simulink model "Power_Model_Official_Pars"  (R2023a)
settings: Solver=ode23t  StartTime=0.0  StopTime=1000  FixedStep=0.01  MaxStep=0.01  RelTol=1e-3  AbsTol=1e-3
values from neighbouring files (symbols this model uses):
  anode_tube_D = 0.01    [fuel_cell_battery_par.mat]
  cathode_tube_D = 0.05    [fuel_cell_battery_par.mat]
  comp_rpm_TLU = [0 1800 3600]    [fuel_cell_battery_par.mat]
  coolant_num_layers = 20    [fuel_cell_battery_par.mat]
  coolant_num_passes = 12    [fuel_cell_battery_par.mat]
  coolant_tube_D = 0.05    [fuel_cell_battery_par.mat]
  coolant_w_channels = 1    [fuel_cell_battery_par.mat]
  env_p = 0.101325    [fuel_cell_battery_par.mat]
  env_T = 20    [fuel_cell_battery_par.mat]
  env_yH20 = 0.0115436377169    [fuel_cell_battery_par.mat]
  env_yO2 = 0.21    [fuel_cell_battery_par.mat]
  radiator_air_area_fins = 11.5625    [fuel_cell_battery_par.mat]
  radiator_air_area_primary = 1.223125    [fuel_cell_battery_par.mat]
  radiator_eta_fin = 0.7    [fuel_cell_battery_par.mat]
  radiator_N_tubes = 25    [fuel_cell_battery_par.mat]
  radiator_rho = 2700    [fuel_cell_battery_par.mat]
  radiator_t_wall = 0.0001    [fuel_cell_battery_par.mat]
  radiator_tube_H = 0.0015    [fuel_cell_battery_par.mat]
  radiator_W = 0.025    [fuel_cell_battery_par.mat]
  stack_area = 280    [fuel_cell_battery_par.mat]
  stack_iL = 1.4    [fuel_cell_battery_par.mat]
  stack_mea_rho = 1800    [fuel_cell_battery_par.mat]
  stack_num_cells = 400    [fuel_cell_battery_par.mat]
  stack_num_channels = 8    [fuel_cell_battery_par.mat]
  stack_t_gdl = 250    [fuel_cell_battery_par.mat]
  stack_t_membrane = 125    [fuel_cell_battery_par.mat]
  stack_w_channels = 1    [fuel_cell_battery_par.mat]
undefined symbols (not defined in the file or in its folder): Bat, f_fc_auxpower, f_fc_currcmd_bpt, f_fc_h2flow, f_fc_heatflow, f_fc_tmpcmd_bpt, f_fc_voltage, Mot, N2_T
libraries: fl_lib x170, nesl_utility x78, FuelCell_lib x32, simulink x5, slpidlib x4, ee_lib x3, autolibshared x1, batteryecm_lib x1, simulink_extras x1
(part 4 of 9)

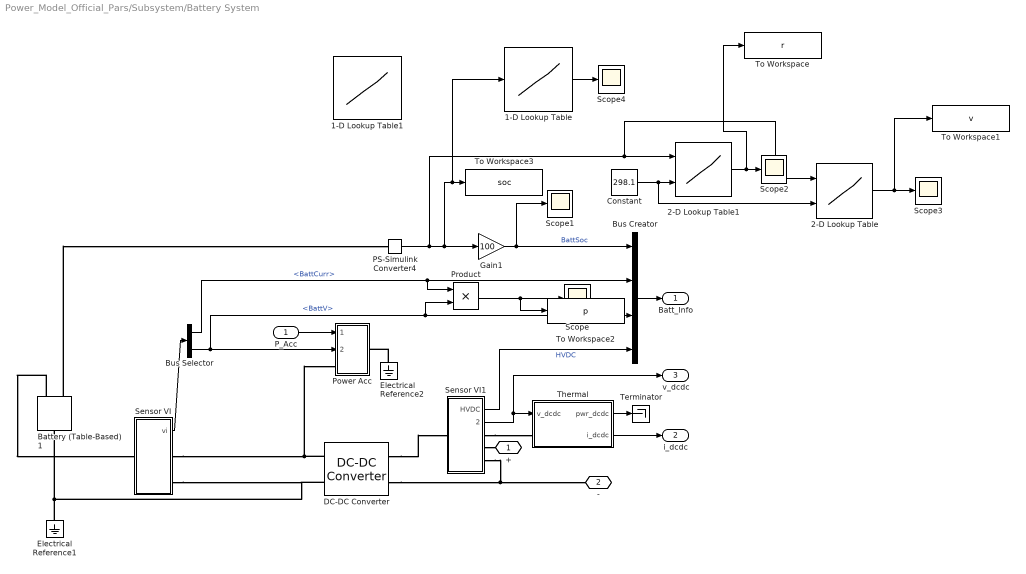
== system Power_Model_Official_Pars/Subsystem/Battery System ==
  P_Acc : Inport
  1-D Lookup Table : Lookup_n-D  NumberOfTableDimensions=1  BreakpointsForDimension1=|  IndexSearchMethod=Linear search  Table=|  ExtrapMethod=Clip  UseLastTableValue=on  InternalRulePriority=Speed  RndMeth=Simplest
      BreakpointsForDimension1=|
      | [0.200266196912653
      | 0.208703993443662
      | 0.217082158618762
      | 0.225401147932810
      | 0.233661407473458
      | 0.241863374201597
      | 0.250007476220565
      | 0.258094133034692
      | 0.266123755797699
      | 0.274096747551458
      | 0.282013503455571
      | 0.289874411008216
      | 0.297679850258674
      | 0.305430194011883
      | 0.313125808025436
      | 0.320767051200107
      | 0.328354275760887
      | 0.335887827433726
      | 0.343368045619003
      | 0.350795263562739
      | 0.358169809006629
      | 0.365492002225901
      | 0.372762157540920
      | 0.379980604257750
      | 0.387147663219995
      | 0.394263583481661
      | 0.401328845877270
      | 0.408344807259339
      | 0.415312528633151
      | 0.422232177852414
      | 0.429103921869992
      | 0.435927926732909
      | 0.442704357577685
      | 0.449433378625998
      | 0.456115153180668
      | 0.462749843621933
      | 0.469337611404045
      | 0.475878617052130
      | 0.482373020159354
      | 0.488820979384337
      | 0.495222652448848
      | 0.501578196135747
      | 0.507887766287174
      | 0.514151517802985
      | 0.520369604639409
      | 0.526542179807939
      | 0.532669395374436
      | 0.538751402458431
      | 0.544788351232696
      | 0.550780390922972
      | 0.556727669807170
      | 0.562630335217596
      | 0.568488533530473
      | 0.574302410199744
      | 0.580072109717100
      | 0.585797772346718
      | 0.591479540262522
      | 0.597117565243885
      | 0.602710710150421
      | 0.608256553325338
      | 0.613754051013394
      | 0.619203525910865
      | 0.624605294684209
      | 0.629959668123070
      | 0.635266951288040
      | 0.640527443653388
      | 0.645741439244992
      | 0.650909226773650
      | 0.656031089763978
      | 0.661107306679072
      | 0.666138151041100
      | 0.671123891547999
      | 0.676064792186425
      | 0.680961112341104
      | 0.685813106900738
      | 0.690621026360585
      | 0.695385116921850
      | 0.700105620588011
      | 0.704782775258189
      | 0.709416814817689
      | 0.714007969225799
      | 0.718556464600965
      | 0.723062523303430
      | 0.727526364015437
      | 0.731948201819075
      | 0.736328248271866
      | 0.740666711480160
      | 0.744963796170435
      | 0.749219703758548
      | 0.753434632417049
      | 0.757608777140570
      | 0.761742329809332
      | 0.765835479251445
      | 0.769888411303126
      | 0.773901308859363
      | 0.777874351956835
      | 0.781807718120983
      | 0.785701580794767
      | 0.789556112063642
      | 0.793371492233416
      | 0.797147876670597
      | 0.800885457679393
      | 0.804584556002125
      | 0.808245419955624
      | 0.811868165288415
      | 0.815452907369891
      | 0.818999761410582
      | 0.822508841965610
      | 0.825980262919708
      | 0.829414137942514
      | 0.832810580234303
      | 0.836169702509582
      | 0.839491616981221
      | 0.842776435345101
      | 0.846024268765268
      | 0.849235227859599
      | 0.852409422685936
      | 0.855546962728712
      | 0.858647956886038
      | 0.861712513457244
      | 0.864740740130864
      | 0.867732743973058
      | 0.870688631416451
      | 0.873608508249394
      | 0.876492479605619
      | 0.879340649954288
      | 0.882153123090427
      | 0.884930002125727
      | 0.887671389479714
      | 0.890377386871260
      | 0.893048095310450
      | 0.895683615090770
      | 0.898284045781626
      | 0.900849486221171
      | 0.903380034509446
      | 0.905875788001805
      | 0.908336843302639
      | 0.910763296259371
      | 0.913155241956721
      | 0.915512774711237
      | 0.917835988066077
      | 0.920124974786031
      | 0.922379826852788
      | 0.924600635460429
      | 0.926787491011139
      | 0.928940483111134
      | 0.931059700566797
      | 0.933145231381011
      | 0.935197162749684
      | 0.937215581058461
      | 0.939200571879608
      | 0.941152219969077
      | 0.943070609263730
      | 0.944955822878720
      | 0.946807943105026
      | 0.948627051407141
      | 0.950413228420884
      | 0.952166553951363
      | 0.953887106971052
      | 0.955574965618005
      | 0.957230207194170
      | 0.958852908163831
      | 0.960443144152144
      | 0.962000989943780
      | 0.963526519481665
      | 0.965019805865805
      | 0.966480921352206
      | 0.967909937351863
      | 0.969306924429842
      | 0.970671952304415
      | 0.972005089846284
      | 0.973306405077848
      | 0.974575965172545
      | 0.975813836454237
      | 0.977020084396656
      | 0.978194773622891
      | 0.979337967904918
      | 0.980449730163172
      | 0.981530122466154
      | 0.982579206030066
      | 0.983597041218479
      | 0.984583687542026
      | 0.985539203658110
      | 0.986463647370639
      | 0.987357075629767
      | 0.988219544531654
      | 0.989051109318228
      | 0.989851824376957
      | 0.990621743240620
      | 0.991360918587080
      | 0.992069402239049
      | 0.992747245163854
      | 0.993394497473180
      | 0.994011208422821
      | 0.994597426412395
      | 0.995153198985054
      | 0.995678572827171
      | 0.996173593768005
      | 0.996638306779337
      | 0.997072755975081
      | 0.997476984610863
      | 0.997851035083571
      | 0.998194948930862
      | 0.998508766830640
      | 0.998792528600487
      | 0.999046273197057
      | 0.999270038715417
      | 0.999463862388352
      | 0.999627780585612
      | 0.999761828813125
      | 0.999866041711916
      | 0.999940453056607
      | 0.999985095757034
      | 1]
      Table=|
      | [0.915178430306573
      | 0.915783431884107
      | 0.916384815525709
      | 0.916982631193170
      | 0.917576910465976
      | 0.918167701856371
      | 0.918755035750723
      | 0.919338959283408
      | 0.919919501712604
      | 0.920496708861588
      | 0.921070608920803
      | 0.921641246464602
      | 0.922208648671976
      | 0.922772858927231
      | 0.923333903451378
      | 0.923891824478798
      | 0.924446647357235
      | 0.924998413187657
      | 0.925547146556990
      | 0.926092887190151
      | 0.926635648451000
      | 0.927175511138715
      | 0.927712463461129
      | 0.928246355386142
      | 0.928777480549568
      | 0.929306139075949
      | 0.929760356358904
      | 0.929908963171485
      | 0.930061992167328
      | 0.930219518390774
      | 0.930381388003597
      | 0.930547676230170
      | 0.930718229418527
      | 0.930893122954263
      | 0.931072203414922
      | 0.931255546328092
      | 0.931442998543326
      | 0.931634635710573
      | 0.931830304993149
      | 0.932030082143342
      | 0.932233814679248
      | 0.932441578435094
      | 0.932653221324051
      | 0.932868819241510
      | 0.933088220535308
      | 0.933311501140874
      | 0.933538509879509
      | 0.933769322705686
      | 0.934003788950851
      | 0.934241984566960
      | 0.934483759447274
      | 0.934729189477170
      | 0.934978125427411
      | 0.935230642138761
      | 0.935486592259489
      | 0.935746120902246
      | 0.936008947807438
      | 0.936275056272835
      | 0.936650959706827
      | 0.937139152070038
      | 0.937625668632281
      | 0.938110624866761
      | 0.938593939245966
      | 0.939075725508591
      | 0.939555902992559
      | 0.940034583734641
      | 0.940511687943600
      | 0.940987325984901
      | 0.941461418943296
      | 0.941934075541715
      | 0.942405217745837
      | 0.942874952663087
      | 0.943343203144841
      | 0.943810074708412
      | 0.944275491095511
      | 0.944739556257189
      | 0.945202194830031
      | 0.945663509221213
      | 0.946123424966667
      | 0.946582042950703
      | 0.947039289613026
      | 0.947495264334783
      | 0.947949894463863
      | 0.948403277896709
      | 0.948855342893808
      | 0.949306185884178
      | 0.949755736045342
      | 0.950204088355061
      | 0.950651172912376
      | 0.951097083258712
      | 0.951541750419461
      | 0.951985266515757
      | 0.952427563492581
      | 0.952868732060419
      | 0.953308705271042
      | 0.953747571863310
      | 0.954185258979779
      | 0.954621891900594
      | 0.955057336405839
      | 0.955491696423272
      | 0.955925005449826
      | 0.956274995551112
      | 0.956366600470192
      | 0.956467188032247
      | 0.956576589847080
      | 0.956694765632499
      | 0.956821541729741
      | 0.956956888252118
      | 0.957100631621624
      | 0.957252731683578
      | 0.957413020203946
      | 0.957581457045985
      | 0.957757874330942
      | 0.957942231958012
      | 0.958134362526053
      | 0.958334225985490
      | 0.958541655531146
      | 0.958756611177275
      | 0.958978926829040
      | 0.959208562574434
      | 0.959445353139352
      | 0.959689258692783
      | 0.959940114887758
      | 0.960197881978899
      | 0.960462396648822
      | 0.960733619239831
      | 0.961011387562640
      | 0.961295662046761
      | 0.961586281725611
      | 0.961883207112953
      | 0.962186278555673
      | 0.962495456646404
      | 0.962810583132458
      | 0.963131618677609
      | 0.963458406512812
      | 0.963790907362966
      | 0.964128966022207
      | 0.964472543264332
      | 0.964821485522594
      | 0.965175753605321
      | 0.965535195657291
      | 0.965899772504938
      | 0.966269334073524
      | 0.966643841189185
      | 0.967023145623261
      | 0.967407208181294
      | 0.967795882543013
      | 0.968189129471260
      | 0.968586804613280
      | 0.968988868665376
      | 0.969395179298334
      | 0.969805697116444
      | 0.970220281867053
      | 0.970638894035402
      | 0.971061395495506
      | 0.971487746585052
      | 0.971917811352010
      | 0.972351549956620
      | 0.972788828665369
      | 0.973229607429851
      | 0.973673754777001
      | 0.974121230417346
      | 0.974571905177660
      | 0.975025738493846
      | 0.975482603529457
      | 0.975942459411147
      | 0.976405181673840
      | 0.976870729099334
      | 0.977338979626243
      | 0.977809891654992
      | 0.978283345558029
      | 0.978759299317056
      | 0.979237635766398
      | 0.979718312430926
      | 0.980201214632876
      | 0.980686299401480
      | 0.981173454570995
      | 0.981662636635579
      | 0.982153735963762
      | 0.982646708474639
      | 0.983141447091491
      | 0.983637907117858
      | 0.984135984050546
      | 0.984635632536609
      | 0.985136750663527
      | 0.985639292380552
      | 0.986143158381420
      | 0.986648301875941
      | 0.987154626178191
      | 0.987662083716622
      | 0.988170580438297
      | 0.988680067948174
      | 0.989190454837568
      | 0.989701691845628
      | 0.990213690217869
      | 0.990726399785184
      | 0.991239734455965
      | 0.991753643110315
      | 0.992268042326961
      | 0.992782879992633
      | 0.993298075362679
      | 0.993813575287865
      | 0.994329301705318
      | 0.994845200387273
      | 0.995361195956707
      | 0.995877233064821
      | 0.996393239023458
      | 0.996909157320446
      | 0.997424917958380
      | 0.997940463218930
      | 0.998455725804436
      | 0.998970646768895
      | 0.999485161417345
      | 1]
  1-D Lookup Table1 : Lookup_n-D  NumberOfTableDimensions=1  BreakpointsForDimension1=|  IndexSearchMethod=Linear search  Table=|  ExtrapMethod=Clip  UseLastTableValue=on  InternalRulePriority=Speed  RndMeth=Simplest
      BreakpointsForDimension1=|
      | [0
      | 0.000580113563438039
      | 0.00122256177108681
      | 0.00190823959853958
      | 0.00263698064198481
      | 0.00340860025465859
      | 0.00422290740215319
      | 0.00507970472367165
      | 0.00597878867169859
      | 0.00691994971764231
      | 0.00790297252323585
      | 0.00892763611470162
      | 0.00999371405938994
      | 0.0111009746442111
      | 0.0122491810558315
      | 0.0134380915622106
      | 0.0146674596952457
      | 0.0159370344342303
      | 0.0172465603898549
      | 0.0185957779884833
      | 0.0199844236564416
      | 0.0214122300040674
      | 0.0228789260092719
      | 0.0243842372003791
      | 0.0259278858380101
      | 0.0275095910957949
      | 0.0291290692396976
      | 0.0307860338057560
      | 0.0324801957760401
      | 0.0342112637526499
      | 0.0359789441295773
      | 0.0377829412622700
      | 0.0396229576347452
      | 0.0414986940241087
      | 0.0434098496623471
      | 0.0453561223952692
      | 0.0473372088384833
      | 0.0493528045303072
      | 0.0514026044784217
      | 0.0534863025070130
      | 0.0556035914107301
      | 0.0577541638883882
      | 0.0599377122715069
      | 0.0621539286627921
      | 0.0644025050654014
      | 0.0666831335085118
      | 0.0689955061695653
      | 0.0713393154927109
      | 0.0737142543036752
      | 0.0761200159209826
      | 0.0785562943243917
      | 0.0810227841327016
      | 0.0835191807126095
      | 0.0860451803974628
      | 0.0886004805110577
      | 0.0911847794613948
      | 0.0937977768267327
      | 0.0964391734381908
      | 0.0991086714589433
      | 0.101805974459993
      | 0.104530787492609
      | 0.107282817157470
      | 0.110061771670563
      | 0.112867360925903
      | 0.115699296555120
      | 0.118557291983989
      | 0.121441062485948
      | 0.124350325232688
      | 0.127284799341860
      | 0.130244205921982
      | 0.133228268114604
      | 0.136236711133805
      | 0.139269262303084
      | 0.142325651089728
      | 0.145405609136705
      | 0.148508870292175
      | 0.151635170636676
      | 0.154784248508053
      | 0.157955844524206
      | 0.161149701603726
      | 0.164365564984480
      | 0.167603182240224
      | 0.170862303295297
      | 0.174142680437480
      | 0.177444068329069
      | 0.180766224016237
      | 0.184108906936746
      | 0.187471878926071
      | 0.190854904221998
      | 0.194257749467758
      | 0.197680183713750
      | 0.201123828234323
      | 0.204594199198603
      | 0.208095049789343
      | 0.211626326245593
      | 0.215187974829860
      | 0.218779941883933
      | 0.222402173727145
      | 0.226054616690707
      | 0.229737217120726
      | 0.233449921379053
      | 0.237192675845071
      | 0.240965426917291
      | 0.244768121014941
      | 0.248600704579532
      | 0.252463124076394
      | 0.256355325996197
      | 0.260277256856452
      | 0.264228863202982
      | 0.268210091611384
      | 0.272220888688462
      | 0.276261201073638
      | 0.280330975440352
      | 0.284430158497430
      | 0.288558696990441
      | 0.292716537703031
      | 0.296903627458234
      | 0.301119913119769
      | 0.305365341593316
      | 0.309639859827769
      | 0.313943414816477
      | 0.318275953598456
      | 0.322637423259597
      | 0.327027770933841
      | 0.331446943804346
      | 0.335894889104629
      | 0.340371554119694
      | 0.344876886187143
      | 0.349410832698267
      | 0.353973341099121
      | 0.358564358891580
      | 0.363183833634381
      | 0.367831712944148
      | 0.372507944496396
      | 0.377212476026522
      | 0.381945255330783
      | 0.386706230267251
      | 0.391495348756754
      | 0.396312558783807
      | 0.401157605733499
      | 0.406029576878204
      | 0.410927736368809
      | 0.415852006770949
      | 0.420802310987588
      | 0.425778554065962
      | 0.430780649663352
      | 0.435808511816117
      | 0.440862054263855
      | 0.445941190801430
      | 0.451045835204430
      | 0.456175901243060
      | 0.461331302683475
      | 0.466511953292056
      | 0.471717766839562
      | 0.476948657105110
      | 0.482204537880173
      | 0.487485322972535
      | 0.492790926210215
      | 0.498121261445356
      | 0.503476242558084
      | 0.508855783460331
      | 0.514259798099629
      | 0.519688200462866
      | 0.525140904580008
      | 0.530617824527790
      | 0.536118874433369
      | 0.541643968477945
      | 0.547193020900342
      | 0.552765946000565
      | 0.558362658143304
      | 0.563983071761421
      | 0.569627101359388
      | 0.575294661516695
      | 0.580985666891219
      | 0.586700032222561
      | 0.592437672335343
      | 0.598198502142466
      | 0.603981980695753
      | 0.609787361680086
      | 0.615614355059884
      | 0.621462875668403
      | 0.627332840133842
      | 0.633224166978663
      | 0.639136773815796
      | 0.645070578388493
      | 0.651025498819906
      | 0.657001453479376
      | 0.662998361004697
      | 0.669016140302906
      | 0.675054710550465
      | 0.681113991193644
      | 0.687193901948879
      | 0.693294362803076
      | 0.699415294013891
      | 0.705556616109995
      | 0.711718249891309
      | 0.717900116429213
      | 0.724102137066739
      | 0.730324233418736
      | 0.736566327372012
      | 0.742828341085456
      | 0.749110196990141
      | 0.755411817789397
      | 0.761733126458873
      | 0.768074046246572
      | 0.774434500672868
      | 0.780814413530505
      | 0.787213708884570
      | 0.793632311072458
      | 0.800070095243506
      | 0.806522428064629
      | 0.812984714183244
      | 0.819456855961407
      | 0.825938756840995
      | 0.832430321329502
      | 0.838931455031139
      | 0.845442064616439
      | 0.851962057811794
      | 0.858491343387172
      | 0.865029831144784
      | 0.871577431907617
      | 0.878134057508083
      | 0.884699620776716
      | 0.891274035530968
      | 0.897857216564068]
      Table=|
      | [0.995764434225388
      | 0.995480710456853
      | 0.995195527656793
      | 0.994910794075989
      | 0.994624399375083
      | 0.994338466450806
      | 0.994050676183280
      | 0.993763359519244
      | 0.993473993985856
      | 0.993185113805298
      | 0.992893998154744
      | 0.992603379630740
      | 0.992310343981287
      | 0.992017817356710
      | 0.991722696909303
      | 0.991428097601730
      | 0.991130732738921
      | 0.990833901431157
      | 0.990534137801466
      | 0.990234920517796
      | 0.989932609105774
      | 0.989630857274062
      | 0.989325854456259
      | 0.989021424956105
      | 0.988713592543245
      | 0.988406347740550
      | 0.988095553006262
      | 0.987785360774595
      | 0.987471476471149
      | 0.987158210200387
      | 0.986841114561938
      | 0.986524653154710
      | 0.986204229888595
      | 0.985884457745113
      | 0.985560596011806
      | 0.985237403003679
      | 0.984909991455063
      | 0.984583273372225
      | 0.984252223473503
      | 0.983921880299489
      | 0.983587091772504
      | 0.983253029773686
      | 0.982914413187848
      | 0.982576543661180
      | 0.982234014791450
      | 0.981892254233096
      | 0.981545733985284
      | 0.981200004012446
      | 0.980849417244870
      | 0.980499645004025
      | 0.980144924319930
      | 0.979791040929682
      | 0.979432121530268
      | 0.979074063434812
      | 0.978710885887283
      | 0.978348594288309
      | 0.977981103833783
      | 0.977614524581627
      | 0.977242671030626
      | 0.976871754517873
      | 0.976495492142971
      | 0.976120193195293
      | 0.975739480621251
      | 0.975359758386117
      | 0.974974558478034
      | 0.974590376311699
      | 0.974200656061629
      | 0.973811981414829
      | 0.973417711827301
      | 0.973024516130069
      | 0.972625672106898
      | 0.972227930652861
      | 0.971824490877610
      | 0.971422182708132
      | 0.971014129530550
      | 0.970607237319017
      | 0.970194556639772
      | 0.969783066576311
      | 0.969365747732268
      | 0.968949649409172
      | 0.968527685059481
      | 0.968106971357551
      | 0.967680357370762
      | 0.967255024346798
      | 0.966823759689191
      | 0.966393806464795
      | 0.965957893090121
      | 0.965523321741994
      | 0.965082764482757
      | 0.964692133397018
      | 0.964398491807232
      | 0.964109738312544
      | 0.963818144508124
      | 0.963531465028549
      | 0.963241928523596
      | 0.962957331699532
      | 0.962669863665839
      | 0.962387358686734
      | 0.962101969487226
      | 0.961821565388891
      | 0.961538265214119
      | 0.961259970878276
      | 0.960978769741420
      | 0.960702593902513
      | 0.960423501643831
      | 0.960149452893033
      | 0.959872479184291
      | 0.959600565973472
      | 0.959325720322327
      | 0.959055950967979
      | 0.958783242722318
      | 0.958515625409440
      | 0.958245063761681
      | 0.957979606547625
      | 0.957711200538970
      | 0.957447911357250
      | 0.957181669881898
      | 0.956920556545957
      | 0.956656488355275
      | 0.956397558562211
      | 0.956135672268859
      | 0.955878933603118
      | 0.955619237685134
      | 0.955364697622162
      | 0.955107200427004
      | 0.954854866336856
      | 0.954599576085403
      | 0.954349455236324
      | 0.954096380026831
      | 0.953848479588790
      | 0.953597627400810
      | 0.953351954449001
      | 0.953103333147255
      | 0.952859894665562
      | 0.952613512003776
      | 0.952372314888201
      | 0.952128178512899
      | 0.951853424448562
      | 0.951459842763293
      | 0.951069104576120
      | 0.950672836393418
      | 0.950279418700638
      | 0.949880647843923
      | 0.949484648401991
      | 0.949083268725806
      | 0.948684679435771
      | 0.948280691037944
      | 0.947879506029189
      | 0.947472905514028
      | 0.947069121057114
      | 0.946659905767869
      | 0.946253518981678
      | 0.945841687057821
      | 0.945432695862774
      | 0.945018246236239
      | 0.944606649345765
      | 0.944189581731073
      | 0.943775378642102
      | 0.943355693526625
      | 0.942938884509769
      | 0.942516583143828
      | 0.942097169233361
      | 0.941672253620132
      | 0.941250236603786
      | 0.940822709489021
      | 0.940398091897601
      | 0.939967956759166
      | 0.939540741856000
      | 0.939108002893245
      | 0.938678194663463
      | 0.938242856786432
      | 0.937810459926094
      | 0.937372528744575
      | 0.936937548649650
      | 0.936497030462084
      | 0.936188548855606
      | 0.935934864789967
      | 0.935686298772107
      | 0.935434344457569
      | 0.935187532514229
      | 0.934937377221564
      | 0.934692320445772
      | 0.934443937031161
      | 0.934200634040847
      | 0.933954020776075
      | 0.933712467986278
      | 0.933467623213128
      | 0.933227818216409
      | 0.932984739839743
      | 0.932746680198154
      | 0.932505366082304
      | 0.932269049331348
      | 0.932029497301101
      | 0.931794920951310
      | 0.931557128793586
      | 0.931324290331989
      | 0.931088255797599
      | 0.930857152689135
      | 0.930622873494519
      | 0.930393503183420
      | 0.930160977012340
      | 0.929933336923488
      | 0.929702561428692
      | 0.929476648968945
      | 0.929247621773797
      | 0.929023434333294
      | 0.928796153033372
      | 0.928564878163429
      | 0.927526871274985
      | 0.926489013853625
      | 0.925444120937927
      | 0.924399540420616
      | 0.923348013507821
      | 0.922296958644185
      | 0.921239046792000
      | 0.920181763656771
      | 0.919117713505793
      | 0.918054445537870
      | 0.916984501013739
      | 0.915915488900236
      | 0.914839891097678
      | 0.913765372669296
      | 0.912684359748886
      | 0.911604569881914
      | 0.910518376974903]
  2-D Lookup Table : Lookup_n-D  BreakpointsForDimension1="[0\t0.200000000000000\t0.400000000000000\t0.600000000000000\t0.800000000000000\t1]"  BreakpointsForDimension2="[243.100000000000\t253.100000000000\t263.100000000000\t273.100000000000\t283.100000000000\t298.100000000000\t313.100000000000]"  Table=|  InternalRulePriority=Speed  RndMeth=Simplest
      | [201.600000000000	201.600000000000	201.600000000000	201.600000000000	201.600000000000	201.600000000000	201.600000000000
      | 258.768000000000	258.768000000000	258.768000000000	258.768000000000	258.768000000000	258.768000000000	258.768000000000
      | 264.960000000000	264.960000000000	264.960000000000	264.960000000000	264.960000000000	264.960000000000	264.960000000000
      | 272.952000000000	272.952000000000	272.952000000000	272.952000000000	272.952000000000	272.952000000000	272.952000000000
      | 286.128000000000	286.128000000000	286.128000000000	286.128000000000	286.128000000000	286.128000000000	286.128000000000
      | 303.912000000000	303.912000000000	303.912000000000	303.912000000000	303.912000000000	303.912000000000	303.912000000000]
      settings: InputPortMap=u0,u1
  2-D Lookup Table1 : Lookup_n-D  BreakpointsForDimension1="[0\t0.200000000000000\t0.400000000000000\t0.600000000000000\t0.800000000000000\t1]"  BreakpointsForDimension2="[243.100000000000\t253.100000000000\t263.100000000000\t273.100000000000\t283.100000000000\t298.100000000000\t313.100000000000]"  Table=|  InternalRulePriority=Speed  RndMeth=Simplest
      | [0.636912000000000	0.460008000000000	0.314208000000000	0.146232000000000	0.103896000000000	0.0403416000000000	0.0740160000000000
      | 0.670968000000000	0.471888000000000	0.295272000000000	0.184536000000000	0.131400000000000	0.0517824000000000	0.0963360000000000
      | 0.649944000000000	0.399816000000000	0.292320000000000	0.182304000000000	0.129240000000000	0.0495864000000000	0.0720000000000000
      | 0.609840000000000	0.397800000000000	0.248544000000000	0.177120000000000	0.128016000000000	0.0544104000000000	0.110592000000000
      | 0.743040000000000	0.435096000000000	0.276912000000000	0.195552000000000	0.138528000000000	0.0529560000000000	0.111312000000000
      | 0.946080000000000	0.561960000000000	0.325224000000000	0.219384000000000	0.160848000000000	0.0730080000000000	0.200808000000000]
      settings: InputPortMap=u0,u1
  Battery (Table-Based)1 : batteryecm_lib/Battery (Table-Based)  SOC_vec=Bat.CapSOCBp  T_dependence=simscape.enum.tablebattery.temperature_dependence.yes  prm_dir=simscape.enum.tablebattery.prm_dir.noCurrentDirectionality  T_vec=Bat.BattTempBp K  V0_mat=Bat.noLoadV V  V0_vec=[3.5057, 3.566, 3.6337, 3.7127, 3.9259, 4.0777, 4.1928] V  V_range=[0.5*min(min(Bat.noLoadV)), 2*max(max(Bat.noLoadV))] V  R0_mat=Bat.R0 Ohm  R0_vec=[.0085, .0085, .0087, .0082, .0083, .0085, .0085] Ohm  R0_dis_mat=[.0117, .0085, .009; .011, .0085, .009; .0114, .0087, .0092; .0107, .0082, .0088; .0107, .0083, .0091; .0113, .0085, .0089; .0116, .0085, .0089] Ohm  R0_dis_vec=[.0085, .0085, .0087, .0082, .0083, .0085, .0085] Ohm  R0_ch_mat=[.0117, .0085, .009; .011, .0085, .009; .0114, .0087, .0092; .0107, .0082, .0088; .0107, .0083, .0091; .0113, .0085, .0089; .0116, .0085, .0089] Ohm  R0_ch_vec=[.0085, .0085, .0087, .0082, .0083, .0085, .0085] Ohm  AH=Bat.AH A*hr  prm_leak=simscape.enum.tablebattery.prm_leak.disabled  Rleak_vec=[8000, 7000, 6000] Ohm  Rleak=7e3 Ohm  extrapolation_option=simscape.enum.extrapolation.linear  SOC_port=simscape.enum.tablebattery.enable.yes  prm_dyn=simscape.enum.tablebattery.prm_dyn.off  R1_mat=[.0109, .0029, .0013; .0069, .0024, .0012; .0047, .0026, .0013; .0034, .0016, .001; .0033, .0023, .0014; .0033, .0018, .0011; .0028, .0017, .0011] Ohm  R1_vec=[.0029, .0024, .0026, .0016, .0023, .0018, .0017] Ohm  tau1_mat=[20, 36, 39; 31, 45, 39; 109, 105, 61; 36, 29, 26; 59, 77, 67; 40, 33, 29; 25, 39, 33] s  tau1_vec=[36, 45, 105, 29, 77, 33, 39] s  R2_mat=[.0109, .0029, .0013; .0069, .0024, .0012; .0047, .0026, .0013; .0034, .0016, .001; .0033, .0023, .0014; .0033, .0018, .0011; .0028, .0017, .0011] Ohm  R2_vec=[.0029, .0024, .0026, .0016, .0023, .0018, .0017] Ohm  tau2_mat=[20, 36, 39; 31, 45, 39; 109, 105, 61; 36, 29, 26; 59, 77, 67; 40, 33, 29; 25, 39, 33] s  tau2_vec=[36, 45, 105, 29, 77, 33, 39] s  R3_mat=[.0109, .0029, .0013; .0069, .0024, .0012; .0047, .0026, .0013; .0034, .0016, .001; .0033, .0023, .0014; .0033, .0018, .0011; .0028, .0017, .0011] Ohm  R3_vec=[.0029, .0024, .0026, .0016, .0023, .0018, .0017] Ohm  tau3_mat=[20, 36, 39; 31, 45, 39; 109, 105, 61; 36, 29, 26; 59, 77, 67; 40, 33, 29; 25, 39, 33] s  tau3_vec=[36, 45, 105, 29, 77, 33, 39] s  R4_mat=[.0109, .0029, .0013; .0069, .0024, .0012; .0047, .0026, .0013; .0034, .0016, .001; .0033, .0023, .0014; .0033, .0018, .0011; .0028, .0017, .0011] Ohm  R4_vec=[.0029, .0024, .0026, .0016, .0023, .0018, .0017] Ohm  tau4_mat=[20, 36, 39; 31, 45, 39; 109, 105, 61; 36, 29, 26; 59, 77, 67; 40, 33, 29; 25, 39, 33] s  tau4_vec=[36, 45, 105, 29, 77, 33, 39] s  R5_mat=[.0109, .0029, .0013; .0069, .0024, .0012; .0047, .0026, .0013; .0034, .0016, .001; .0033, .0023, .0014; .0033, .0018, .0011; .0028, .0017, .0011] Ohm  R5_vec=[.0029, .0024, .0026, .0016, .0023, .0018, .0017] Ohm  tau5_mat=[20, 36, 39; 31, 45, 39; 109, 105, 61; 36, 29, 26; 59, 77, 67; 40, 33, 29; 25, 39, 33] s  tau5_vec=[36, 45, 105, 29, 77, 33, 39] s  prm_fade=simscape.enum.tablebattery.prm_fade.disabled  N0=100  dV0=0  dR0=0  dAH=0  dRleak=0  dR1=0  dR2=0  dR3=0  dR4=0  dR5=0  N0vec=[100, 200, 300]  Tfadevec=[298.15, 323.15] K  dV0vec=[0, 0, 0]  dR0vec=[0, 0, 0]  dAHvec=[0, 0, 0]  dRleakvec=[0, 0, 0]  dR1vec=[0, 0, 0]  dR2vec=[0, 0, 0]  dR3vec=[0, 0, 0]  dR4vec=[0, 0, 0]  dR5vec=[0, 0, 0]  dV0mat=[0, 0; 0, 0; 0, 0]  dR0mat=[0, 0; 0, 0; 0, 0]  dAHmat=[0, 0; 0, 0; 0, 0]  dRleakmat=[0, 0; 0, 0; 0, 0]  dR1mat=[0, 0; 0, 0; 0, 0]  dR2mat=[0, 0; 0, 0; 0, 0]  dR3mat=[0, 0; 0, 0; 0, 0]  dR4mat=[0, 0; 0, 0; 0, 0]  dR5mat=[0, 0; 0, 0; 0, 0]  prm_age_modeling=simscape.enum.tablebattery.prm_age_modeling.equation  storage_dt_age_vec=[0] d  storage_T_age_vec=[273] K  prm_age_OCV=simscape.enum.tablebattery.prm_age_OCV.OCV  OCV_age=0.9  SOC_age=0.6  prm_age_resistance=simscape.enum.tablebattery.prm_age.disabled  OCV_scaling_age_resistance=2.2134e6  OCV_offset_age_resistance=1.632e6  temp_exp_age_resistance=0.515833569 V  t_exp_age_resistance=0.75  T_age_vec_resistance=[273.15, 298.15, 323.15] K  dt_age_vec_resistance=[90, 180, 270, 360] d  dR0_age_vec=[0, 0, 0]  t_meas_dR0_age=100 d  dR0_age_mat=[0, 0, 0; 0, 0, 0; 0, 0, 0; 0, 0, 0]  prm_age_capacity=simscape.enum.tablebattery.prm_age.disabled  OCV_scaling_age_capacity=1.5097e07  OCV_offset_age_capacity=8.3625e06  temp_exp_age_capacity=0.6011 V  t_exp_age_capacity=0.75  T_age_vec_capacity=[273.15, 298.15, 323.15] K  dt_age_vec_capacity=[90, 180, 270, 360] d  dAH_age_vec=[0, 0, 0]  t_meas_dAH_age=100 d  dAH_age_mat=[0, 0, 0; 0, 0, 0; 0, 0, 0; 0, 0, 0]  thermal_port=simscape.enum.thermaleffects.omit  temperature=298.15 K  thermal_mass=Bat.thermalMass J/K  i_specify=off  i_priority=None  i=0 A  i_nominal_specify=off  i_nominal_unit=A  i_nominal_value=1  v_specify=off  v_priority=None  v=0 V  v_nominal_specify=off  v_nominal_unit=V  v_nominal_value=1  stateOfCharge_specify=on  stateOfCharge_priority=High  stateOfCharge=0  stateOfCharge_nominal_specify=off  stateOfCharge_nominal_unit=1  stateOfCharge_nominal_value=1  num_cycles_specify=off  num_cycles_priority=High  num_cycles=0  num_cycles_nominal_specify=off  num_cycles_nominal_unit=1  num_cycles_nominal_value=1  cell_temperature_specify=off  cell_temperature_priority=High  cell_temperature=298.15 K  cell_temperature_nominal_specify=off  cell_temperature_nominal_unit=K  cell_temperature_nominal_value=1
      settings: InternalSimscapePortConfiguration="{\"Bottom\":[],\"Left\":[{\"id\":\"p\",\"label\":\"+\",\"type\":\"foundation.electrical.electrical\"},{\"id\":\"soc\",\"label\":\"SOC\",\"type\":\"output\"}],\"Right\":[{\"id\":\"n\",\"label\":\"-\",\"type\":\"foundation.electrical.electrical\"}],\"Top\":[]}"
  Bus Creator : BusCreator  Inputs=4
  Bus Selector : BusSelector  OutputSignals=BattCurr,BattV
  Constant : Constant  Value=298.1
  DC-DC Converter : ee_lib/Semiconductors & Converters/Converters/DC-DC Converter  Vref_option=ee.enum.converters.voltageref.internal  v_ref=BattDCDC.Vout V  P_rated=200 kW  droop_enabled=true  droop_param=ee.enum.converters.droop.value  droop=0.1 V/A  droop_percent=2  Vref_droop=10 V  reversible=ee.enum.converters.directionality.bidirectional  G_diode=1e-8 1/Ohm  P_fixed=1 W  losses_option=ee.enum.converters.lossesOption.proportionalToSquaredCurrent  eff_rated=95  tableOption=ee.enum.converters.lossTableOption.current  i_eff_vec=[1, 2, 3, 4] A  v_eff_vec=[15, 30, 45] V  eff_vec=[90, 80, 70, 60]  eff_2D_table=[90, 85, 80; 80, 75, 70; 70, 65, 60; 60, 55, 50]  model_dynamics=ee.enum.converters.dynamics.no  tau=0.02 s  v_ini=10 V  v1_min=1 V  R1=1000 Ohm  R2=1000 Ohm  enable_fault=simscape.enum.onoff.off  fault_condition=ee.enum.faults.faultInputCondition.greaterThan  fault_threshold=0.5  T_eff_vec=[280, 300, 320] K  eff_3D_table=repmat([66; 76; 80; 74], 1, 3, 3)  thermal_mass=100 J/K  initial_temperature=298.15 K
      settings: InternalSimscapePortConfiguration="{\"Bottom\":[],\"Left\":[{\"id\":\"p1\",\"label\":\"1+\",\"type\":\"foundation.electrical.electrical\"},{\"id\":\"n1\",\"label\":\"1-\",\"type\":\"foundation.electrical.electrical\"}],\"Right\":[{\"id\":\"p2\",\"label\":\"2+\",\"type\":\"foundation.electrical.electrical\"},{\"id\":\"n2\",\"label\":\"2-\",\"type\":\"foundation.electrical.electrical\"}],\"Top\":[]}"
  Electrical Reference1 : fl_lib/Electrical/Electrical Elements/Electrical Reference
  Electrical Reference2 : fl_lib/Electrical/Electrical Elements/Electrical Reference
  Gain1 : Gain  Gain=100
  PS-Simulink Converter4 : nesl_utility/PS-Simulink Converter  PhysicalDomain=network_engine_domain  SubClassName=ps_output  LeftPortType=input  RightPortType=output  PseudoPeriodic=off  Frequencies=[]  VectorFormat=1-D array  Unit=1  AffineConversion=off
  Power Acc : Subsystem
  Product : Product
  Scope{,1..4} (5 alike) : Scope
  Sensor VI : Subsystem
  Sensor VI1 : Subsystem
  Terminator : Terminator
  Thermal : Subsystem
  To Workspace : ToWorkspace  VariableName=r  SampleTime=1
  To Workspace1 : ToWorkspace  VariableName=v  SampleTime=1
  To Workspace2 : ToWorkspace  VariableName=p  SampleTime=1
  To Workspace3 : ToWorkspace  VariableName=soc  SampleTime=1
  + : PMIOPort  Side=Right
  - : PMIOPort  Port=2  Side=Right
  Batt_Info : Outport
  i_dcdc : Outport  Port=2
  v_dcdc : Outport  Port=3
  wires:
  Bus Selector/1 -> Product/1, Bus Creator/2  "<BattCurr>"
  PS-Simulink Converter4/1 -> 2-D Lookup Table/1, 2-D Lookup Table1/1, 1-D Lookup Table/1, To Workspace3/1, Gain1/1
  Sensor VI/1(vi) -> Bus Selector/1
  Gain1/1 -> Scope1/1, Bus Creator/1  "BattSoc"
  Bus Selector/2 -> Product/2, Bus Creator/3, Power Acc/2(VBatt)  "<BattV>"
  Sensor VI1/1(HVDC) -> Bus Creator/4  "HVDC"
  P_Acc/1 -> Power Acc/1(P_Acc)
  Bus Creator/1 -> Batt_Info/1
  Sensor VI1/2(v_dcdc) -> Thermal/1(v_dcdc), v_dcdc/1
  Thermal/2(i_dcdc) -> i_dcdc/1
  Thermal/1(pwr_dcdc) -> Terminator/1
  Product/1 -> To Workspace2/1, Scope/1
  Constant/1 -> 2-D Lookup Table/2, 2-D Lookup Table1/2
  2-D Lookup Table1/1 -> To Workspace/1, Scope2/1
  2-D Lookup Table/1 -> To Workspace1/1, Scope3/1
  1-D Lookup Table/1 -> Scope4/1
  connections:
  Battery (Table-Based)1/LConn2 -- PS-Simulink Converter4/LConn1
  Electrical Reference2/LConn1 -- Power Acc/RConn1
  Battery (Table-Based)1/LConn1 -- Sensor VI/LConn1
  Sensor VI1/RConn2 -- +/RConn1
  Sensor VI1/RConn1 -- Thermal/LConn1
  Sensor VI/RConn1 -- DC-DC Converter/LConn1 -- Power Acc/LConn1
  DC-DC Converter/RConn1 -- Sensor VI1/LConn1
  Sensor VI1/RConn3 -- -/RConn1 -- DC-DC Converter/RConn2
  Electrical Reference1/LConn1 -- Sensor VI/RConn2 -- DC-DC Converter/LConn2 -- Battery (Table-Based)1/RConn1

== system Power_Model_Official_Pars/Subsystem/Electrical Load9 ==
  Controlled Current Source : fl_lib/Electrical/Electrical Sources/Controlled Current Source
  Electrical Reference : fl_lib/Electrical/Electrical Elements/Electrical Reference
  Inputs : Subsystem  Variant=on  VariantControlMode=label  LabelModeActiveChoice=Ramp
      settings: PortSchema="{\"entries\":[{\"content\":{\"sides\":[{\"content\":{\"connectorIds\":[\"LConn1\"]},\"type\":\"ConnectorPlacement.EquallySpacedRectSide\",\"uuid\":\"316ab41f-9548-4c29-941b-82cd3006a9cc\"},{\"content\":{\"side\":\"RIGHT\"},\"type\":\"ConnectorPlacement.EquallySpacedRectSide\",\"uuid\":\"21ddf6a1-5f8a-47a4-ab15-3c27c3a556ce\"},{\"content\":{\"connectorIds\":[\"LConn2\"],\"side\":\"TOP\"},\"type\":\"ConnectorPlacement.EquallySpacedRectSide\",\"uuid\":\"59191a52-f145-4ac2-9cf2-0e0b54b3d2a8\"}]},\"type\":\"ConnectorPlacement.EquallySpacedConnector\",\"uuid\":\"e8f988fd-b412-4b1a-aaea-374cf82170cc\"}],\"packageUris\":[\"http://schema.mathworks.com/mf0/Connector/R2020b\"],\"version\":\"1.0\"}"
      mask Display:
      | blk = get_param(gcb, 'CompiledActiveChoiceBlock');
      | eval(get_param(blk, 'MaskDisplay'))
  Voltage Sensor : fl_lib/Electrical/Electrical Sensors/Voltage Sensor
  - : PMIOPort  Side=Right
  + : PMIOPort  Port=2  Side=Right
  connections:
  Voltage Sensor/RConn1 -- Inputs/LConn2
  Inputs/LConn1 -- Controlled Current Source/RConn1
  Controlled Current Source/RConn2 -- Voltage Sensor/LConn1 -- +/RConn1
  Voltage Sensor/RConn2 -- -/RConn1 -- Controlled Current Source/LConn1 -- Electrical Reference/LConn1

== system Power_Model_Official_Pars/氢气罐/Pressure-Reducing Valve ==
  Absolute Reference (MA) : fl_lib/Moist Air/Elements/Absolute Reference (MA)
  PS Add : fl_lib/Physical Signals/Functions/PS Add
  PS Constant : fl_lib/Physical Signals/Sources/PS Constant  constant=r_max^2
  PS Constant1 : fl_lib/Physical Signals/Sources/PS Constant  constant=p_range MPa
  PS Gain : fl_lib/Physical Signals/Functions/PS Gain  gain=(r_min^2 - r_max^2)/p_range 1/MPa
  PS Gain1 : fl_lib/Physical Signals/Functions/PS Gain  gain=pi*D^2/4 m^2
  PS Subtract : fl_lib/Physical Signals/Functions/PS Subtract
  PS Subtract1 : fl_lib/Physical Signals/Functions/PS Subtract
  Pressure & Temperature Sensor (MA) : fl_lib/Moist Air/Sensors/Pressure & Temperature Sensor (MA)  reference=foundation.enum.MeasurementReference.difference  pressure=true  pressure_spec=foundation.enum.PressureMeasementSpec.Absolute  temperature=true
      settings: InternalSimscapePortConfiguration="{\"Bottom\":[{\"id\":\"T\",\"label\":\"T\",\"type\":\"output\"}],\"Left\":[{\"id\":\"A\",\"label\":\"A\",\"type\":\"foundation.moist_air.moist_air\"}],\"Right\":[{\"id\":\"B\",\"label\":\"B\",\"type\":\"foundation.moist_air.moist_air\"},{\"id\":\"P\",\"label\":\"P\",\"type\":\"output\"}],\"Top\":[]}"
  Valve : fl_lib/Moist Air/Elements/Local Restriction (MA)  restriction_type=foundation.enum.restriction_type.variable  restriction_area=0.001 m^2  min_area=pi*(r_min*D)^2/4 m^2  max_area=pi*(r_max*D)^2/4 m^2  area=pi*D^2/4 m^2  Cd=0.64  B_lam=0.999
  A : PMIOPort  Side=Left
  B : PMIOPort  Port=2  Side=Right
  p_set : PMIOPort  Port=3  Side=Left
  connections:
  Valve/LConn1 -- A/RConn1
  Valve/RConn1 -- B/RConn1 -- Pressure & Temperature Sensor (MA)/LConn1
  Absolute Reference (MA)/LConn1 -- Pressure & Temperature Sensor (MA)/RConn1
  PS Gain1/RConn1 -- Valve/LConn2
  Pressure & Temperature Sensor (MA)/RConn2 -- PS Subtract/LConn1
  PS Gain/LConn1 -- PS Subtract/RConn1
  PS Add/RConn1 -- PS Gain1/LConn1
  PS Add/LConn2 -- PS Gain/RConn1
  PS Constant/RConn1 -- PS Add/LConn1
  PS Subtract1/RConn1 -- PS Subtract/LConn2
  PS Subtract1/LConn1 -- p_set/RConn1
  PS Constant1/RConn1 -- PS Subtract1/LConn2

== system Power_Model_Official_Pars/氧气供给(压缩机)/Sensors ==
  Abs : Abs  ZeroCross=off  SaturateOnIntegerOverflow=off
  Average Efficiency : fl_lib/Physical Signals/Sources/PS Constant  constant=0.5
  PS Divide : fl_lib/Physical Signals/Functions/PS Divide
  PS Product : fl_lib/Physical Signals/Functions/PS Product
  PS-Simulink Converter : nesl_utility/PS-Simulink Converter  PhysicalDomain=network_engine_domain  SubClassName=ps_output  LeftPortType=input  RightPortType=output  PseudoPeriodic=off  Frequencies=[]  VectorFormat=1-D array  Unit=inherit  AffineConversion=off
  PS-Simulink Converter1 : nesl_utility/PS-Simulink Converter  PhysicalDomain=network_engine_domain  SubClassName=ps_output  LeftPortType=input  RightPortType=output  PseudoPeriodic=off  Frequencies=[]  VectorFormat=inherit  Unit=inherit  AffineConversion=off
  Pressure & Temperature Sensor (MA) : fl_lib/Moist Air/Sensors/Pressure & Temperature Sensor (MA)  reference=foundation.enum.MeasurementReference.difference  pressure=true  pressure_spec=foundation.enum.PressureMeasementSpec.Absolute  temperature=true
      settings: InternalSimscapePortConfiguration="{\"Bottom\":[{\"id\":\"T\",\"label\":\"T\",\"type\":\"output\"}],\"Left\":[{\"id\":\"A\",\"label\":\"A\",\"type\":\"foundation.moist_air.moist_air\"}],\"Right\":[{\"id\":\"B\",\"label\":\"B\",\"type\":\"foundation.moist_air.moist_air\"},{\"id\":\"P\",\"label\":\"P\",\"type\":\"output\"}],\"Top\":[]}"
  Volumetric Flow Rate Sensor (MA) : fl_lib/Moist Air/Sensors/Flow Rate Sensor (MA)  mass_flow_measure=false  volumetric_flow_measure=true  volumetric_flow_conditions=foundation.enum.volumetric_flow_conditions.actual  p_std=0.101325 MPa  T_std=20 degC  RH_std=0.65  energy_flow_measure=false  vapor_flow_measure=false  gas_flow_measure=false
      settings: InternalSimscapePortConfiguration="{\"Bottom\":[],\"Left\":[{\"id\":\"A\",\"label\":\"A\",\"type\":\"foundation.moist_air.moist_air\"}],\"Right\":[{\"id\":\"B\",\"label\":\"B\",\"type\":\"foundation.moist_air.moist_air\"},{\"id\":\"V\",\"label\":\"V\",\"type\":\"output\"}],\"Top\":[]}"
  A_P : PMIOPort  Side=Left
  A : PMIOPort  Port=2  Side=Left
  B : PMIOPort  Port=3  Side=Right
  Power : Outport
  tag scope: p_o2=global
  wires:
  PS-Simulink Converter/1 -> Abs/1
  Abs/1 -> Power/1
  PS-Simulink Converter1/1 -> [p_o2]
  connections:
  Volumetric Flow Rate Sensor (MA)/RConn1 -- Pressure & Temperature Sensor (MA)/RConn1 -- B/RConn1
  Pressure & Temperature Sensor (MA)/RConn2 -- PS-Simulink Converter1/LConn1 -- PS Product/LConn1
  Volumetric Flow Rate Sensor (MA)/RConn2 -- PS Product/LConn2
  PS Divide/LConn1 -- PS Product/RConn1
  Average Efficiency/RConn1 -- PS Divide/LConn2
  PS-Simulink Converter/LConn1 -- PS Divide/RConn1
  Pressure & Temperature Sensor (MA)/LConn1 -- A_P/RConn1
  Volumetric Flow Rate Sensor (MA)/LConn1 -- A/RConn1

== system Power_Model_Official_Pars/氧气供给(压缩机)/压缩机控制 ==
  OER : Inport
  i : Inport  Port=2
  M_meas : Inport  Port=3
  Constant : Constant  Value=0.1 * stack_iL * stack_area
  Control Signals : Scope  NumInputPorts=2
  M_set : Gain  Gain=stack_num_cells * 32e-3 / (4*96485) /0.2095
  Max : MinMax  Function=max  Inputs=2  ZeroCross=off
  Mux : Mux  Inputs=2
  Mux1 : Mux  Inputs=2
  PID Controller : slpidlib/PID Controller  Controller=PI  Form=Ideal  TimeDomain=Continuous-time  UseExternalTs=off  SampleTime=-1  IntegratorMethod=Forward Euler  FilterMethod=Forward Euler  ControllerParametersSource=internal  P=5  I=0.5  UseKiTs=off  D=0  N=100  UseFilter=on  TunerSelectOption=Transfer Function Based (PID Tuner App)  InitialConditionSource=internal  InitialConditionForIntegrator=0  InitialConditionForFilter=0  DifferentiatorICPrevScaledInput=0  ExternalReset=none  TrackingMode=off  Kt=1  LimitOutput=on  SatLimitsSource=internal  UpperSaturationLimit=1  LowerSaturationLimit=0  LinearizeAsGain=on  AntiWindupMode=back-calculation  Kb=1  LimitIntegrator=off  UpperIntegratorSaturationLimit=inf  LowerIntegratorSaturationLimit=-inf  POutMin=[]  POutMax=[]  IOutMin=[]  IOutMax=[]  DOutMin=[]  DOutMax=[]  NOutMin=[]  NOutMax=[]  SumOutMin=[]  SumOutMax=[]  SaturationOutMin=[]  SaturationOutMax=[]  PParamMin=[]  PParamMax=[]  IParamMin=[]  IParamMax=[]  DParamMin=[]  DParamMax=[]  NParamMin=[]  NParamMax=[]  KbParamMin=[]  KbParamMax=[]  KtParamMin=[]  KtParamMax=[]  KbOutMin=[]  KbOutMax=[]  KtOutMin=[]  KtOutMax=[]  IntegratorOutMin=[]  IntegratorOutMax=[]  FilterOutMin=[]  FilterOutMax=[]  SumI1OutMin=[]  SumI1OutMax=[]  SumI2OutMin=[]  SumI2OutMax=[]  SumI3OutMin=[]  SumI3OutMax=[]  SumI4OutMin=[]  SumI4OutMax=[]  SumDOutMin=[]  SumDOutMax=[]  DifferentiatorOutMin=[]  DifferentiatorOutMax=[]  FilterDiffOutCoefMin=[]  FilterDiffOutCoefMax=[]  ReciprocalOutMin=[]  ReciprocalOutMax=[]  SumDenOutMin=[]  SumDenOutMax=[]  SumNumOutMin=[]  SumNumOutMax=[]  DivideOutMin=[]  DivideOutMax=[]  UdiffTsProdOutMin=[]  UdiffTsProdOutMax=[]  NTsProdOutMin=[]  NTsProdOutMax=[]  UintegralTsProdOutMin=[]  UintegralTsProdOutMax=[]  UngainTsProdOutMin=[]  UngainTsProdOutMax=[]  ClampingZeroOutDataTypeStr=Inherit: Inherit via back propagation  ClampingZeroOutMin=[]  ClampingZeroOutMax=[]  FilterDenConstantOutDataTypeStr=Inherit: Inherit via back propagation  FilterDenConstantOutMin=[]  FilterDenConstantOutMax=[]  PCopyOutDataTypeStr=Inherit: Inherit via back propagation  PCopyOutMin=[]  PCopyOutMax=[]  NCopyOutDataTypeStr=Inherit: Inherit via back propagation  NCopyOutMin=[]  NCopyOutMax=[]  IntegratorContinuousStateAttributes=''  IntegratorStateMustResolveToSignalObject=off  IntegratorRTWStateStorageClass=Auto  FilterContinuousStateAttributes=''  FilterStateMustResolveToSignalObject=off  FilterRTWStateStorageClass=Auto  ParallelPVariant=Passthrough  IdealPVariant=InternalParameters  IVariant=InternalParameters  DVariant=Disabled  IntegratorVariant=Continuous  SatVariant=Enabled  AWVariant=BackCalculation  PCopyVariant=Disabled  TRVariant=Disabled  FdbkBlocksVariant=Forward  IdealPFdbkVariant=Disabled  SatFdbkVariant=Disabled  DerivativeFilterVariant=Disabled  NVariant=Disabled  NCopyVariant=Disabled_SignalSpec  FilterICVariant=Disabled  IntegratorICVariant=InternalICs  ExternalResetVariant=Disabled  TRSumVariant=Passthrough  SumFdbkVariant=Disabled  SumVariant=Sum_PI  TsampFilterVariant=InternalTs  TsampNgainVariant=Passthrough  TsampIntegralVariant=Disabled_SignalSpec  ExternalSaturationOutDataTypeStr=Inherit: Same as second input
  Product : Product
  Sum : Sum  Inputs=|+-
  Transfer Fcn : TransferFcn  Denominator=[2 1]
  cmd : Outport
  wires:
  Mux1/1 -> Control Signals/2
  Mux/1 -> Control Signals/1
  Transfer Fcn/1 -> cmd/1, Mux1/2
  M_meas/1 -> Sum/2, Mux/2
  Product/1 -> M_set/1
  M_set/1 -> Mux/1, Sum/1
  Sum/1 -> PID Controller/1
  PID Controller/1 -> Transfer Fcn/1, Mux1/1
  Max/1 -> Product/2
  i/1 -> Max/1
  Constant/1 -> Max/2
  OER/1 -> Product/1
